simulink model "Motor_sim"  (R2017a)
settings: Solver=VariableStepAuto  StartTime=0.0  StopTime=1  FixedStep=0.001  RelTol=1e-3
values from neighbouring files (symbols this model uses):
  B = 0.0050681847    [RunSim.m]
  J = 0.0012822507    [RunSim.m]
  Kb = 0.722435011    [RunSim.m]
  Km = 0.722435011    [RunSim.m]
  L = 4.5371111111*10^-3    (= 0.0045371111111)    [RunSim.m]
  R = 5.39166    [RunSim.m]
  sample_time = 0.005    [RunSim.m]
undefined symbols (not defined in the file or in its folder): DiscIntNeverNeededParam, sigbuilder_block
libraries: simulink x1, fuzblock x1
settings Model: Creator=daniel  LastModifiedBy=chi
settings OptimizationCC: LifeSpan=inf
settings DebuggingCC: SFExecutionAtInitializationDiag=none

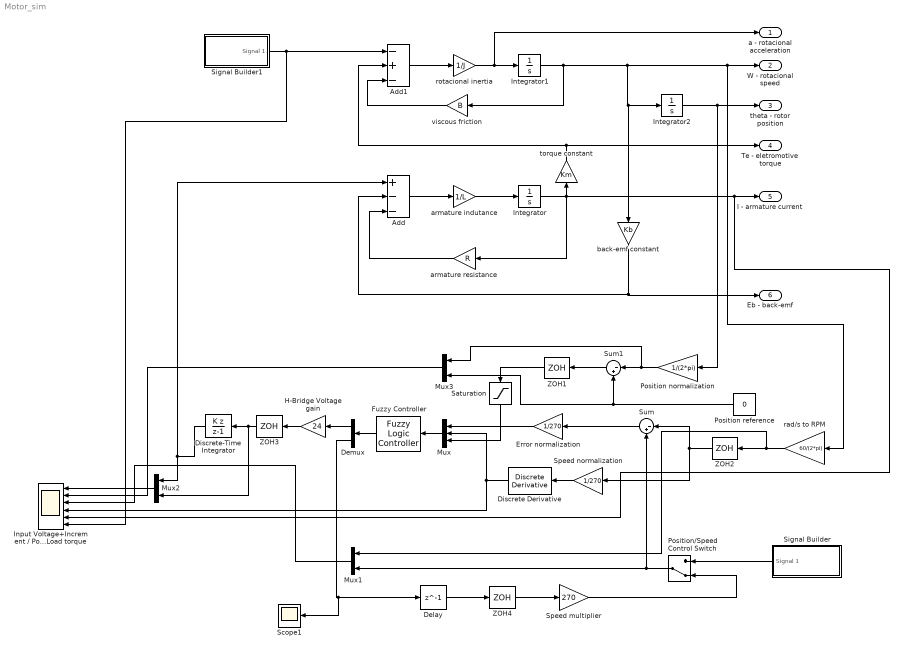
== system Motor_sim ==
  Add : Sum  Inputs=+--
  Add1 : Sum  Inputs=-+-
  Delay : Delay  DelayLength=1  InitialCondition=0  SampleTime=sample_time
  Demux : Demux  Outputs=2
  Discrete Derivative : simulink/Discrete/Discrete Derivative  gainval=1.0  ICPrevScaledInput=0.0  OutMin=[]  OutMax=[]  OutDataType=fixdt(1, 16)  OutScaling=2^-10  DoSatur=off
  Discrete-Time Integrator : DiscreteIntegrator  IntegratorMethod=Accumulation: Backward Euler  InitialConditionSetting=State (most efficient)  SampleTime=sample_time  LimitOutput=on  UpperSaturationLimit=24  LowerSaturationLimit=-24  ICPrevOutput=DiscIntNeverNeededParam  ICPrevScaledInput=DiscIntNeverNeededParam
  Error normalization : Gain  Gain=1/270
  Fuzzy Controller : fuzblock/Fuzzy Logic  Controller  fis=fuzzy_controller
  H-Bridge Voltage gain : Gain  Gain=24
  Input Voltage+Increment / Position + Ref / Speed + Ref / Acceleration / Current / Load torque : Scope  NumInputPorts=6
  Integrator : Integrator
  Integrator1 : Integrator
  Integrator2 : Integrator
  Mux : Mux  Inputs=3
  Mux1 : Mux  Inputs=2
  Mux2 : Mux  Inputs=2
  Mux3 : Mux  Inputs=2
  Position normalization : Gain  Gain=1/(2*pi)
  Position reference : Constant  Value=0  SampleTime=sample_time
  Position/Speed Control Switch : ManualSwitch  CurrentSetting=0
  Saturation : Saturate  UpperLimit=1  LowerLimit=-1
  Scope1 : Scope
  Signal Builder : Subsystem  Tag=STV Subsys  LoadFcn=sigbuilder_block('load');  StartFcn=sigbuilder_block('start');  StopFcn=sigbuilder_block('stop');  ClipboardFcn=sigbuilder_block('clipboard');  mask(Sigbuilder block){tuvar=[0:10]}
      mask help: Simulink:masks:SigbuilderBlock_MD
      mask init:
      | if ~strcmp(get_param(bdroot(gcbh),'SimulationStatus'),'stopped') tuvar = sigbuilder_block('maskInit'); end
      settings: CopyFcn=sigbuilder_block('copy');  DeleteFcn=sigbuilder_block('delete');  ModelCloseFcn=sigbuilder_block('modelClose');  PreSaveFcn=sigbuilder_block('preSave');  PauseFcn=sigbuilder_block('pause');  ContinueFcn=sigbuilder_block('continue');  NameChangeFcn=sigbuilder_block('namechange');  OpenFcn=sigbuilder_block('open',[320.25 71.25 565.5 444.75 ]);  CloseFcn=sigbuilder_block('close');
      mask Display: plot(0, 0, 100, 100,[2, 2, 32, 32, 2], [68, 8, 8, 68, 68],[32, 2], [38, 38], [32, 19, 2],[53, 60, 44], [32, 17, 17, 2],[16, 16, 31, 31]);txt = getActiveGroup(gcbh);text(2, 100, txt,'verticalAlignment', 'top');
  Signal Builder1 : Subsystem  Tag=STV Subsys  LoadFcn=sigbuilder_block('load',[418.5 0 588 512.25 ]);  StartFcn=sigbuilder_block('start');  StopFcn=sigbuilder_block('stop');  ClipboardFcn=sigbuilder_block('clipboard');  mask(Sigbuilder block){tuvar=[0:10]}
      mask help: Simulink:masks:SigbuilderBlock_MD
      mask init:
      | if ~strcmp(get_param(bdroot(gcbh),'SimulationStatus'),'stopped') tuvar = sigbuilder_block('maskInit'); end
      settings: CopyFcn=sigbuilder_block('copy');  DeleteFcn=sigbuilder_block('delete');  ModelCloseFcn=sigbuilder_block('modelClose');  PreSaveFcn=sigbuilder_block('preSave');  PauseFcn=sigbuilder_block('pause');  ContinueFcn=sigbuilder_block('continue');  NameChangeFcn=sigbuilder_block('namechange');  OpenFcn=sigbuilder_block('open',[418.5 0 588 512.25 ]);  CloseFcn=sigbuilder_block('close');
      mask Display: plot(0, 0, 100, 100,[2, 2, 32, 32, 2], [68, 8, 8, 68, 68],[32, 2], [38, 38], [32, 19, 2],[53, 60, 44], [32, 17, 17, 2],[16, 16, 31, 31]);txt = getActiveGroup(gcbh);text(2, 100, txt,'verticalAlignment', 'top');
  Speed normalization : Gain  Gain=1/270
  Speed multiplier : Gain  Gain=270
  Sum : Sum  Inputs=|-+
  Sum1 : Sum  Inputs=|-+
  ZOH{1..4} (4 alike) : ZeroOrderHold  SampleTime=sample_time
  "armature indutance " : Gain  Gain=1/L
  "armature resistance " : Gain  Gain=R
  back-emf constant : Gain  Gain=Kb
  rad/s to RPM : Gain  Gain=60/(2*pi)
  rotacional inertia : Gain  Gain=1/J
  torque constant : Gain  Gain=Km
  viscous friction : Gain  Gain=B
  a - rotacional acceleration : Outport
  W - rotacional speed : Outport  Port=2
  theta - rotor position : Outport  Port=3
  Te - eletromotive torque : Outport  Port=4
  I - armature current : Outport  Port=5
  Eb - back-emf : Outport  Port=6
  wires:
  Add/1 -> "armature indutance "/1
  "armature indutance "/1 -> Integrator/1
  "armature resistance "/1 -> Add/3
  Integrator/1 -> I - armature current/1, Input Voltage+Increment / Position + Ref / Speed + Ref / Acceleration / Current / Load torque/5, torque constant/1, "armature resistance "/1
  Signal Builder1/1(Signal 1) -> Add1/1, Input Voltage+Increment / Position + Ref / Speed + Ref / Acceleration / Current / Load torque/6
  Add1/1 -> rotacional inertia/1
  rotacional inertia/1 -> a - rotacional acceleration/1, Integrator1/1
  viscous friction/1 -> Add1/3
  Integrator1/1 -> back-emf constant/1, Integrator2/1, rad/s to RPM/1, W - rotacional speed/1, viscous friction/1
  torque constant/1 -> Te - eletromotive torque/1, Add1/2
  Integrator2/1 -> Position normalization/1, theta - rotor position/1
  back-emf constant/1 -> Eb - back-emf/1, Add/2
  H-Bridge Voltage gain/1 -> ZOH3/1
  Sum/1 -> Error normalization/1
  Discrete-Time Integrator/1 -> Add/1, Mux2/1
  ZOH2/1 -> Sum/1, Speed normalization/1
  rad/s to RPM/1 -> Mux1/1, ZOH2/1
  Mux1/1 -> Input Voltage+Increment / Position + Ref / Speed + Ref / Acceleration / Current / Load torque/3
  Speed normalization/1 -> Discrete Derivative/1
  ZOH3/1 -> Mux2/2, Discrete-Time Integrator/1
  Discrete Derivative/1 -> Mux/2, Input Voltage+Increment / Position + Ref / Speed + Ref / Acceleration / Current / Load torque/4
  Mux/1 -> Fuzzy Controller/1
  Error normalization/1 -> Mux/1
  Position reference/1 -> Sum1/2, Mux3/2
  Sum1/1 -> ZOH1/1
  Fuzzy Controller/1 -> Demux/1
  Demux/1 -> H-Bridge Voltage gain/1
  Demux/2 -> Scope1/1, Delay/1
  Position/Speed Control Switch/1 -> Sum/2, Mux1/2
  ZOH4/1 -> Speed multiplier/1
  Delay/1 -> ZOH4/1
  ZOH1/1 -> Saturation/1
  Position normalization/1 -> Mux3/1, Sum1/1
  Speed multiplier/1 -> Position/Speed Control Switch/2
  Saturation/1 -> Mux/3
  Mux2/1 -> Input Voltage+Increment / Position + Ref / Speed + Ref / Acceleration / Current / Load torque/1
  Mux3/1 -> Input Voltage+Increment / Position + Ref / Speed + Ref / Acceleration / Current / Load torque/2
  Signal Builder/1(Signal 1) -> Position/Speed Control Switch/1

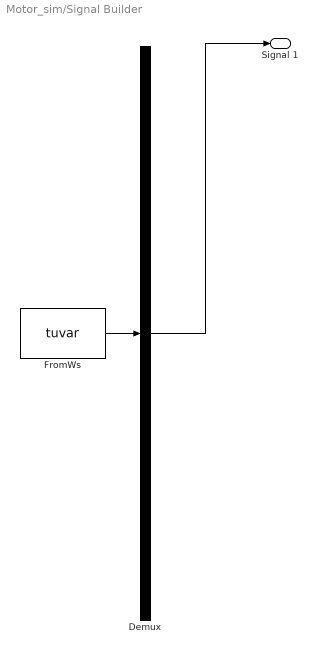
== system Motor_sim/Signal Builder ==
  Demux : Demux  Tag=STV Demux  Outputs=1
  FromWs : FromWorkspace  Tag=STV FromWs  VariableName=tuvar  SampleTime=0
      SigBuilderData=|
      | common.afterFinalStr = 'Extrapolate'
      | common.sampleTime = 0
      | dataSet.timeRange = [0 10]
      | dataSet.name = 'Group 1'
      | sbobj.Groups.Name = 'Group 1'
      | sbobj.Groups.Signals.Name = 'Signal 1'
      | sbobj.Groups.Signals.XData = [0 0.1 0.1 0.2 0.2 0.3 0.45 0.75 0.9 10]
      | sbobj.Groups.Signals.YData = [270 270 -270 -270 0 0 270 -270 0 -3]
  Signal 1 : Outport  Tag=STV Outport
  wires:
  Demux/1 -> Signal 1/1
  FromWs/1 -> Demux/1

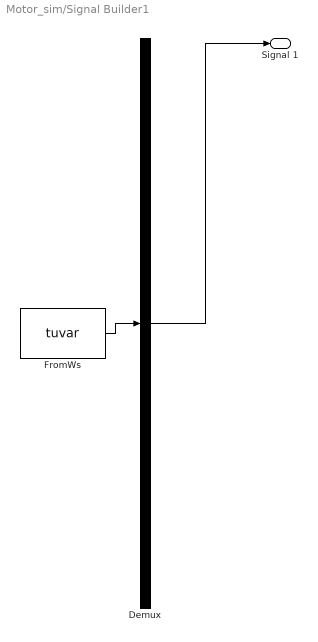
== system Motor_sim/Signal Builder1 ==
  Demux : Demux  Tag=STV Demux  Outputs=1
  FromWs : FromWorkspace  Tag=STV FromWs  VariableName=tuvar  SampleTime=0
      SigBuilderData=|
      | common.afterFinalStr = 'Extrapolate'
      | common.sampleTime = 0
      | dataSet.timeRange = [0 10]
      | dataSet.name = 'Group 1'
      | sbobj.Groups.Name = 'Group 1'
      | sbobj.Groups.Signals.Name = 'Signal 1'
      | sbobj.Groups.Signals.XData = [0 0.5 0.5 1 10]
      | sbobj.Groups.Signals.YData = [2 2 0 0 1.78]
      | sbobj.Groups.TimeRange = [0 10]
  Signal 1 : Outport  Tag=STV Outport
  wires:
  Demux/1 -> Signal 1/1
  FromWs/1 -> Demux/1
